simulink model "RC_model_iden"  (R2023b)
settings: Solver=ode1  StartTime=0.0  StopTime=0.848  FixedStep=0.001  RelTol=1e-3  EnableMultiTasking=on
values from neighbouring files (symbols this model uses):
  a = 0.3    [RC_cal_demo.m]    (also in RC_cal_demo_01.m = 1.19001595204e-05; RC_cal_dongtai.m = 4.75514899903e-06; RC_iden_demo.m = V(1); RC_iden_demo01.m = V(1))
  a1 = 189.2    [RC_cal_demo.m]    (also in RC_cal_demo_01.m = 216.986140272; RC_iden_demo.m = V(2); RC_iden_demo01.m = V(2); RC_iden_dongtai.m = 0)
  a2 = 709.081    [RC_cal_demo.m]    (also in RC_cal_demo_01.m = 51.9969921477; RC_iden_demo.m = V(3); RC_iden_demo01.m = V(3); RC_iden_dongtai.m = 0)
  a3 = 0    [RC_cal_demo.m]    (also in RC_cal_demo_01.m = -4.85038740997; RC_cal_dongtai.m = -4.66745370581; RC_iden_demo.m = V(4); RC_iden_demo01.m = V(4))
  b = 0    [RC_cal_demo.m]    (also in RC_cal_demo_01.m = -4.99998404294; RC_cal_dongtai.m = -5.74572134537; RC_iden_Optimization_fmincon_11canshu.m = []; RC_iden_Optimization_fmincon_dongtai.m = [])
  c1 = 11    [RC_cal_demo.m]    (also in RC_cal_demo_01.m = 3.69821992975; RC_iden_demo.m = V(6); RC_iden_demo01.m = V(6); RC_iden_dongtai.m = 0)
  c2 = 22.7    [RC_cal_demo.m]    (also in RC_cal_demo_01.m = 8.28628350298; RC_iden_demo.m = V(7); RC_iden_demo01.m = V(7); RC_iden_dongtai.m = 0)
  c3 = 0    [RC_cal_demo.m]    (also in RC_cal_demo_01.m = 0.0112779556916; RC_iden_demo.m = V(8); RC_iden_demo01.m = V(8); RC_iden_dongtai.m = V(4))
  f0 = -2.1    [RC_cal_demo.m]    (also in RC_cal_demo_01.m = 4.66079282314; RC_cal_dongtai.m = 4.52749017489; RC_iden_demo.m = V(9); RC_iden_demo01.m = V(9))
  k = 0.3    [RC_cal_demo.m]    (also in RC_cal_demo_01.m = -0.0271829954254; RC_cal_dongtai.m = -0.017999550541; RC_iden_demo.m = V(10); RC_iden_demo01.m = V(10))
  m = 0.0141707256428496    (= 0.0141707256428)    [RC_cal_demo_01.m]    (also in RC_cal_dongtai.m = 0.0195846403036; RC_iden_demo01.m = V(11); RC_iden_dongtai.m = V(7))
settings Model: Creator=lenovo  LastModifiedBy=Lenovo
settings SolverCC: AlgebraicLoopSolver=TrustRegion
settings DataIOCC: ReturnWorkspaceOutputs=off
settings OptimizationCC: LifeSpan=inf
settings DebuggingCC: UnconnectedInputMsg=warning  UnconnectedOutputMsg=warning  UnconnectedLineMsg=warning  SFUnexpectedBacktrackingDiag=warning  SFNoUnconditionalDefaultTransitionDiag=warning  SFExecutionAtInitializationDiag=none  ArithmeticOperatorsInVariantConditions=warning
settings ModelReferenceCC: EnableRefExpFcnMdlSchedulingChecks=on
settings SFSimCC: SimUseLocalCustomCode=off  CustomCodeUndefinedFunction=UseInterfaceOnly
settings RTWCC: RTWUseLocalCustomCode=off
settings CodeAppCC: StateflowObjectComments=on
settings GRTTargetCC: TargetLangStandard=C89/C90 (ANSI)
settings ConfigComp: CovMetricSettings=dw  CovSaveCumulativeToWorkspaceVar=on  CovSaveSingleToWorkspaceVar=on  CovExternalEMLEnable=off

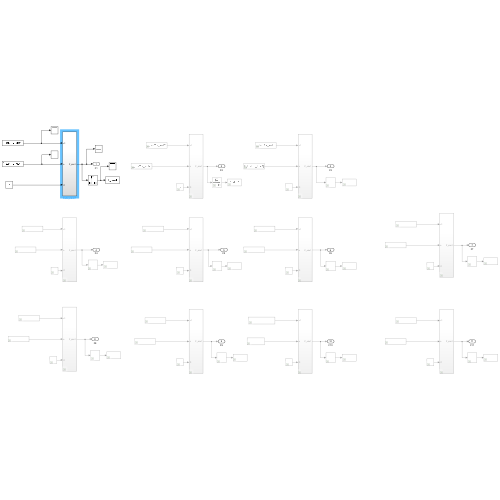
[thumbnail: Simulink's stored preview of the top-level diagram]
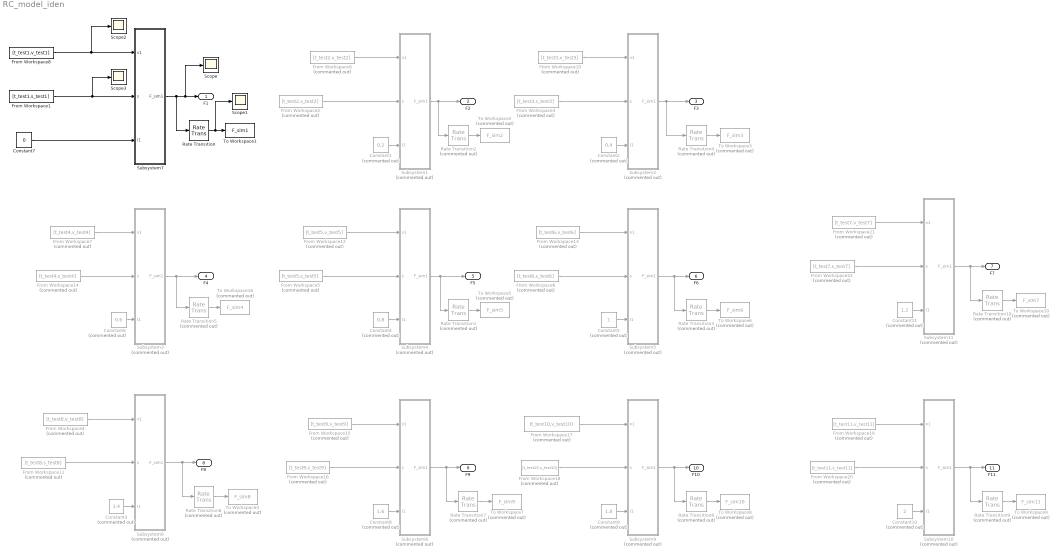
== system RC_model_iden ==
  Constant1 : Constant  Commented=on  Value=0.2
  Constant10 : Constant  Commented=on  Value=2
  Constant11 : Constant  Commented=on  Value=1.2
  Constant2 : Constant  Commented=on  Value=0.4
  Constant3 : Constant  Commented=on  Value=1.4
  Constant4 : Constant  Commented=on  Value=0.8
  Constant5 : Constant  Commented=on
  Constant6 : Constant  Commented=on  Value=0.6
  Constant7 : Constant  Value=0
  Constant8 : Constant  Commented=on  Value=1.6
  Constant9 : Constant  Commented=on  Value=1.8
  From Workspace1 : FromWorkspace  VariableName=[t_test1,s_test1]
  From Workspace10 : FromWorkspace  Commented=on  VariableName=[t_test3,v_test3]
  From Workspace11 : FromWorkspace  Commented=on  VariableName=[t_test8,s_test8]
  From Workspace12 : FromWorkspace  Commented=on  VariableName=[t_test5,v_test5]
  From Workspace13 : FromWorkspace  Commented=on  VariableName=[t_test6,v_test6]
  From Workspace14 : FromWorkspace  Commented=on  VariableName=[t_test4,s_test4]
  From Workspace15 : FromWorkspace  Commented=on  VariableName=[t_test9,v_test9]
  From Workspace16 : FromWorkspace  Commented=on  VariableName=[t_test9,s_test9]
  From Workspace17 : FromWorkspace  Commented=on  VariableName=[t_test10,v_test10]
  From Workspace18 : FromWorkspace  Commented=on  VariableName=[t_test10,s_test10]
  From Workspace19 : FromWorkspace  Commented=on  VariableName=[t_test11,v_test11]
  From Workspace2 : FromWorkspace  Commented=on  VariableName=[t_test2,s_test2]
  From Workspace20 : FromWorkspace  Commented=on  VariableName=[t_test11,s_test11]
  From Workspace21 : FromWorkspace  Commented=on  VariableName=[t_test7,v_test7]
  From Workspace22 : FromWorkspace  Commented=on  VariableName=[t_test7,s_test7]
  From Workspace3 : FromWorkspace  Commented=on  VariableName=[t_test3,s_test3]
  From Workspace4 : FromWorkspace  Commented=on  VariableName=[t_test8,v_test8]
  From Workspace5 : FromWorkspace  Commented=on  VariableName=[t_test5,s_test5]
  From Workspace6 : FromWorkspace  Commented=on  VariableName=[t_test6,s_test6]
  From Workspace7 : FromWorkspace  Commented=on  VariableName=[t_test4,v_test4]
  From Workspace8 : FromWorkspace  VariableName=[t_test1,v_test1]
  From Workspace9 : FromWorkspace  Commented=on  VariableName=[t_test2,v_test2]
  Rate Transition : RateTransition  OutPortSampleTime=0.001
  Rate Transition{1..10} (10 alike) : RateTransition  Commented=on  OutPortSampleTime=0.001
  Scope{,1..3} (4 alike) : Scope
  Subsystem1 : Subsystem  Commented=on
  Subsystem10 : Subsystem  Commented=on
  Subsystem11 : Subsystem  Commented=on
  Subsystem2 : Subsystem  Commented=on
  Subsystem3 : Subsystem  Commented=on
  Subsystem4 : Subsystem  Commented=on
  Subsystem5 : Subsystem  Commented=on
  Subsystem6 : Subsystem  Commented=on
  Subsystem7 : Subsystem
  Subsystem8 : Subsystem  Commented=on
  Subsystem9 : Subsystem  Commented=on
  To Workspace1 : ToWorkspace  VariableName=F_sim1  SampleTime=-1
  To Workspace10 : ToWorkspace  Commented=on  VariableName=F_sim7  SampleTime=-1
  To Workspace16 : ToWorkspace  Commented=on  VariableName=F_sim4  SampleTime=-1
  To Workspace2 : ToWorkspace  Commented=on  VariableName=F_sim2  SampleTime=-1
  To Workspace3 : ToWorkspace  Commented=on  VariableName=F_sim3  SampleTime=-1
  To Workspace4 : ToWorkspace  Commented=on  VariableName=F_sim8  SampleTime=-1
  To Workspace5 : ToWorkspace  Commented=on  VariableName=F_sim5  SampleTime=-1
  To Workspace6 : ToWorkspace  Commented=on  VariableName=F_sim6  SampleTime=-1
  To Workspace7 : ToWorkspace  Commented=on  VariableName=F_sim9  SampleTime=-1
  To Workspace8 : ToWorkspace  Commented=on  VariableName=F_sim10  SampleTime=-1
  To Workspace9 : ToWorkspace  Commented=on  VariableName=F_sim11  SampleTime=-1
  F1 : Outport  VectorParamsAs1DForOutWhenUnconnected=off
  F2 : Outport  Port=2  VectorParamsAs1DForOutWhenUnconnected=off
  F3 : Outport  Port=3  VectorParamsAs1DForOutWhenUnconnected=off
  F4 : Outport  Port=4  VectorParamsAs1DForOutWhenUnconnected=off
  F5 : Outport  Port=5  VectorParamsAs1DForOutWhenUnconnected=off
  F6 : Outport  Port=6  VectorParamsAs1DForOutWhenUnconnected=off
  F7 : Outport  Port=7  VectorParamsAs1DForOutWhenUnconnected=off
  F8 : Outport  Port=8  VectorParamsAs1DForOutWhenUnconnected=off
  F9 : Outport  Port=9  VectorParamsAs1DForOutWhenUnconnected=off
  F10 : Outport  Port=10  VectorParamsAs1DForOutWhenUnconnected=off
  F11 : Outport  Port=11  VectorParamsAs1DForOutWhenUnconnected=off
  wires:
  From Workspace9/1 -> Subsystem1/1(v1)
  Subsystem1/1(F_sim1) -> F2/1, Rate Transition2/1
  From Workspace2/1 -> Subsystem1/2(s)
  Constant1/1 -> Subsystem1/3(I1)
  From Workspace10/1 -> Subsystem2/1(v1)
  Subsystem2/1(F_sim1) -> Rate Transition4/1, F3/1
  From Workspace3/1 -> Subsystem2/2(s)
  Constant2/1 -> Subsystem2/3(I1)
  From Workspace12/1 -> Subsystem4/1(v1)
  Subsystem4/1(F_sim1) -> F5/1, Rate Transition1/1
  From Workspace5/1 -> Subsystem4/2(s)
  Constant4/1 -> Subsystem4/3(I1)
  From Workspace13/1 -> Subsystem5/1(v1)
  Subsystem5/1(F_sim1) -> Rate Transition3/1, F6/1
  From Workspace6/1 -> Subsystem5/2(s)
  Constant5/1 -> Subsystem5/3(I1)
  From Workspace8/1 -> Scope2/1, Subsystem7/1(v1)
  Subsystem7/1(F_sim1) -> Rate Transition/1, Scope/1, F1/1
  From Workspace1/1 -> Scope3/1, Subsystem7/2(s)
  Constant7/1 -> Subsystem7/3(I1)
  Rate Transition/1 -> To Workspace1/1, Scope1/1
  Rate Transition1/1 -> To Workspace5/1
  Rate Transition2/1 -> To Workspace2/1
  Rate Transition3/1 -> To Workspace6/1
  Rate Transition4/1 -> To Workspace3/1
  Rate Transition5/1 -> To Workspace16/1
  Constant6/1 -> Subsystem3/3(I1)
  From Workspace14/1 -> Subsystem3/2(s)
  Subsystem3/1(F_sim1) -> F4/1, Rate Transition5/1
  From Workspace7/1 -> Subsystem3/1(v1)
  Rate Transition6/1 -> To Workspace4/1
  From Workspace11/1 -> Subsystem6/2(s)
  Constant3/1 -> Subsystem6/3(I1)
  From Workspace4/1 -> Subsystem6/1(v1)
  Subsystem6/1(F_sim1) -> Rate Transition6/1, F8/1
  Rate Transition7/1 -> To Workspace7/1
  From Workspace16/1 -> Subsystem8/2(s)
  Constant8/1 -> Subsystem8/3(I1)
  From Workspace15/1 -> Subsystem8/1(v1)
  Subsystem8/1(F_sim1) -> Rate Transition7/1, F9/1
  Rate Transition8/1 -> To Workspace8/1
  From Workspace18/1 -> Subsystem9/2(s)
  Constant9/1 -> Subsystem9/3(I1)
  From Workspace17/1 -> Subsystem9/1(v1)
  Subsystem9/1(F_sim1) -> Rate Transition8/1, F10/1
  Rate Transition9/1 -> To Workspace9/1
  From Workspace20/1 -> Subsystem10/2(s)
  Constant10/1 -> Subsystem10/3(I1)
  From Workspace19/1 -> Subsystem10/1(v1)
  Subsystem10/1(F_sim1) -> Rate Transition9/1, F11/1
  Rate Transition10/1 -> To Workspace10/1
  From Workspace22/1 -> Subsystem11/2(s)
  Constant11/1 -> Subsystem11/3(I1)
  From Workspace21/1 -> Subsystem11/1(v1)
  Subsystem11/1(F_sim1) -> Rate Transition10/1, F7/1

== system RC_model_iden/Subsystem1 ==
  v1 : Inport
  s : Inport  Port=2
  I1 : Inport  Port=3
  Ftra : Subsystem
  Subsystem : Subsystem
  F_sim1 : Outport  VectorParamsAs1DForOutWhenUnconnected=off
  wires:
  s/1 -> Ftra/2(x1), Subsystem/1(x1)
  v1/1 -> Ftra/3(x2)
  I1/1 -> Ftra/1(I)
  Subsystem/1(z) -> Ftra/4(z)
  Ftra/1(Ftra) -> F_sim1/1

== system RC_model_iden/Subsystem10 ==
  v1 : Inport
  s : Inport  Port=2
  I1 : Inport  Port=3
  Ftra : Subsystem
  Subsystem : Subsystem
  F_sim1 : Outport  VectorParamsAs1DForOutWhenUnconnected=off
  wires:
  s/1 -> Ftra/2(x1), Subsystem/1(x1)
  v1/1 -> Ftra/3(x2)
  I1/1 -> Ftra/1(I)
  Subsystem/1(z) -> Ftra/4(z)
  Ftra/1(Ftra) -> F_sim1/1

== system RC_model_iden/Subsystem11 ==
  v1 : Inport
  s : Inport  Port=2
  I1 : Inport  Port=3
  Ftra : Subsystem
  Subsystem : Subsystem
  F_sim1 : Outport  VectorParamsAs1DForOutWhenUnconnected=off
  wires:
  s/1 -> Ftra/2(x1), Subsystem/1(x1)
  v1/1 -> Ftra/3(x2)
  I1/1 -> Ftra/1(I)
  Subsystem/1(z) -> Ftra/4(z)
  Ftra/1(Ftra) -> F_sim1/1

== system RC_model_iden/Subsystem2 ==
  v1 : Inport
  s : Inport  Port=2
  I1 : Inport  Port=3
  Ftra : Subsystem
  Subsystem : Subsystem
  F_sim1 : Outport  VectorParamsAs1DForOutWhenUnconnected=off
  wires:
  s/1 -> Ftra/2(x1), Subsystem/1(x1)
  v1/1 -> Ftra/3(x2)
  I1/1 -> Ftra/1(I)
  Subsystem/1(z) -> Ftra/4(z)
  Ftra/1(Ftra) -> F_sim1/1

== system RC_model_iden/Subsystem3 ==
  v1 : Inport
  s : Inport  Port=2
  I1 : Inport  Port=3
  Ftra : Subsystem
  Subsystem : Subsystem
  F_sim1 : Outport  VectorParamsAs1DForOutWhenUnconnected=off
  wires:
  s/1 -> Ftra/2(x1), Subsystem/1(x1)
  v1/1 -> Ftra/3(x2)
  I1/1 -> Ftra/1(I)
  Subsystem/1(z) -> Ftra/4(z)
  Ftra/1(Ftra) -> F_sim1/1

== system RC_model_iden/Subsystem4 ==
  v1 : Inport
  s : Inport  Port=2
  I1 : Inport  Port=3
  Ftra : Subsystem
  Subsystem : Subsystem
  F_sim1 : Outport  VectorParamsAs1DForOutWhenUnconnected=off
  wires:
  s/1 -> Ftra/2(x1), Subsystem/1(x1)
  v1/1 -> Ftra/3(x2)
  I1/1 -> Ftra/1(I)
  Subsystem/1(z) -> Ftra/4(z)
  Ftra/1(Ftra) -> F_sim1/1

== system RC_model_iden/Subsystem5 ==
  v1 : Inport
  s : Inport  Port=2
  I1 : Inport  Port=3
  Ftra : Subsystem
  Subsystem : Subsystem
  F_sim1 : Outport  VectorParamsAs1DForOutWhenUnconnected=off
  wires:
  s/1 -> Ftra/2(x1), Subsystem/1(x1)
  v1/1 -> Ftra/3(x2)
  I1/1 -> Ftra/1(I)
  Subsystem/1(z) -> Ftra/4(z)
  Ftra/1(Ftra) -> F_sim1/1

== system RC_model_iden/Subsystem6 ==
  v1 : Inport
  s : Inport  Port=2
  I1 : Inport  Port=3
  Ftra : Subsystem
  Subsystem : Subsystem
  F_sim1 : Outport  VectorParamsAs1DForOutWhenUnconnected=off
  wires:
  s/1 -> Ftra/2(x1), Subsystem/1(x1)
  v1/1 -> Ftra/3(x2)
  I1/1 -> Ftra/1(I)
  Subsystem/1(z) -> Ftra/4(z)
  Ftra/1(Ftra) -> F_sim1/1

== system RC_model_iden/Subsystem7 ==
  v1 : Inport
  s : Inport  Port=2
  I1 : Inport  Port=3
  Ftra : Subsystem
  Subsystem : Subsystem
  F_sim1 : Outport  VectorParamsAs1DForOutWhenUnconnected=off
  wires:
  s/1 -> Ftra/2(x1), Subsystem/1(x1)
  v1/1 -> Subsystem/2(v1), Ftra/3(x2)
  I1/1 -> Ftra/1(I)
  Subsystem/1(z) -> Ftra/4(z)
  Ftra/1(Ftra) -> F_sim1/1

== system RC_model_iden/Subsystem8 ==
  v1 : Inport
  s : Inport  Port=2
  I1 : Inport  Port=3
  Ftra : Subsystem
  Subsystem : Subsystem
  F_sim1 : Outport  VectorParamsAs1DForOutWhenUnconnected=off
  wires:
  s/1 -> Ftra/2(x1), Subsystem/1(x1)
  v1/1 -> Ftra/3(x2)
  I1/1 -> Ftra/1(I)
  Subsystem/1(z) -> Ftra/4(z)
  Ftra/1(Ftra) -> F_sim1/1

== system RC_model_iden/Subsystem9 ==
  v1 : Inport
  s : Inport  Port=2
  I1 : Inport  Port=3
  Ftra : Subsystem
  Subsystem : Subsystem
  F_sim1 : Outport  VectorParamsAs1DForOutWhenUnconnected=off
  wires:
  s/1 -> Ftra/2(x1), Subsystem/1(x1)
  v1/1 -> Ftra/3(x2)
  I1/1 -> Ftra/1(I)
  Subsystem/1(z) -> Ftra/4(z)
  Ftra/1(Ftra) -> F_sim1/1

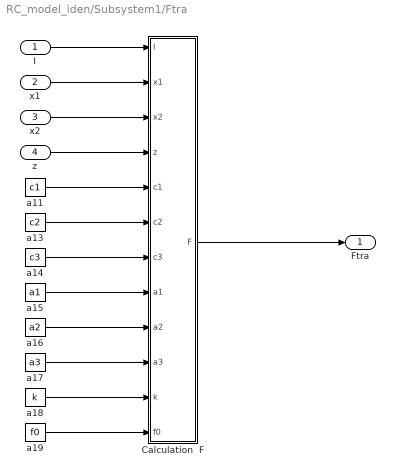
== system RC_model_iden/Subsystem1/Ftra ==
  I : Inport
  x1 : Inport  Port=2
  x2 : Inport  Port=3
  z : Inport  Port=4
  Calculation  F : MATLAB Function  TreatAsAtomicUnit=on
  a11 : Constant  Value=c1  SampleTime=-1
  a13 : Constant  Value=c2  SampleTime=-1
  a14 : Constant  Value=c3  SampleTime=-1
  a15 : Constant  Value=a1  SampleTime=-1
  a16 : Constant  Value=a2  SampleTime=-1
  a17 : Constant  Value=a3  SampleTime=-1
  a18 : Constant  Value=k  SampleTime=-1
  a19 : Constant  Value=f0  SampleTime=-1
  Ftra : Outport  VectorParamsAs1DForOutWhenUnconnected=off
  wires:
  x2/1 -> Calculation  F/3(x2)
  a14/1 -> Calculation  F/7(c3)
  a15/1 -> Calculation  F/8(a1)
  a16/1 -> Calculation  F/9(a2)
  a17/1 -> Calculation  F/10(a3)
  a19/1 -> Calculation  F/12(f0)
  a18/1 -> Calculation  F/11(k)
  a13/1 -> Calculation  F/6(c2)
  a11/1 -> Calculation  F/5(c1)
  Calculation  F/1(F) -> Ftra/1
  z/1 -> Calculation  F/4(z)
  x1/1 -> Calculation  F/2(x1)
  I/1 -> Calculation  F/1(I)

== system RC_model_iden/Subsystem1/Subsystem ==
  x1 : Inport
  Constant : Constant  Value=a
  Constant1 : Constant  Value=b
  Delay : Delay  DelayLength=1  InitialCondition=0
  Delay1 : Delay  DelayLength=1  InitialCondition=0
  Delay2 : Delay  DelayLength=1  InitialCondition=0.17
  Delay3 : Delay  DelayLength=1  InitialCondition=0
  MATLAB Function : MATLAB Function  TreatAsAtomicUnit=on
  z : Outport  VectorParamsAs1DForOutWhenUnconnected=off
  wires:
  Delay3/1 -> MATLAB Function/6(x0)
  MATLAB Function/3(x01) -> Delay3/1
  Delay2/1 -> MATLAB Function/7(S0)
  MATLAB Function/4(S01) -> Delay2/1
  Delay1/1 -> MATLAB Function/5(x1k1)
  MATLAB Function/2(x1k2) -> Delay1/1
  Delay/1 -> MATLAB Function/4(zk1)
  MATLAB Function/1(zk) -> z/1, Delay/1
  Constant1/1 -> MATLAB Function/2(b)
  Constant/1 -> MATLAB Function/1(a)
  x1/1 -> MATLAB Function/3(x1k)

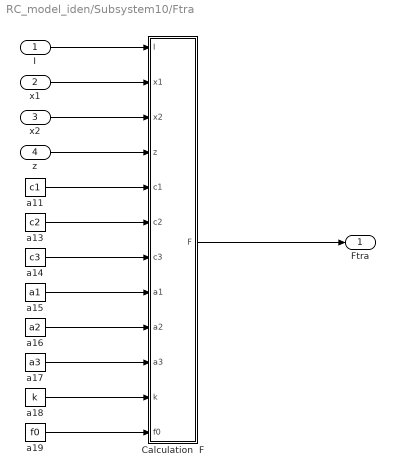
== system RC_model_iden/Subsystem10/Ftra ==
  I : Inport
  x1 : Inport  Port=2
  x2 : Inport  Port=3
  z : Inport  Port=4
  Calculation  F : MATLAB Function  TreatAsAtomicUnit=on
  a11 : Constant  Value=c1  SampleTime=-1
  a13 : Constant  Value=c2  SampleTime=-1
  a14 : Constant  Value=c3  SampleTime=-1
  a15 : Constant  Value=a1  SampleTime=-1
  a16 : Constant  Value=a2  SampleTime=-1
  a17 : Constant  Value=a3  SampleTime=-1
  a18 : Constant  Value=k  SampleTime=-1
  a19 : Constant  Value=f0  SampleTime=-1
  Ftra : Outport  VectorParamsAs1DForOutWhenUnconnected=off
  wires:
  x2/1 -> Calculation  F/3(x2)
  a14/1 -> Calculation  F/7(c3)
  a15/1 -> Calculation  F/8(a1)
  a16/1 -> Calculation  F/9(a2)
  a17/1 -> Calculation  F/10(a3)
  a19/1 -> Calculation  F/12(f0)
  a18/1 -> Calculation  F/11(k)
  a13/1 -> Calculation  F/6(c2)
  a11/1 -> Calculation  F/5(c1)
  Calculation  F/1(F) -> Ftra/1
  z/1 -> Calculation  F/4(z)
  x1/1 -> Calculation  F/2(x1)
  I/1 -> Calculation  F/1(I)

== system RC_model_iden/Subsystem10/Subsystem ==
  x1 : Inport
  Constant : Constant  Value=a
  Constant1 : Constant  Value=b
  Delay : Delay  DelayLength=1  InitialCondition=0
  Delay1 : Delay  DelayLength=1  InitialCondition=0
  Delay2 : Delay  DelayLength=1  InitialCondition=0.17
  Delay3 : Delay  DelayLength=1  InitialCondition=0
  MATLAB Function : MATLAB Function  TreatAsAtomicUnit=on
  z : Outport  VectorParamsAs1DForOutWhenUnconnected=off
  wires:
  Delay3/1 -> MATLAB Function/6(x0)
  MATLAB Function/3(x01) -> Delay3/1
  Delay2/1 -> MATLAB Function/7(S0)
  MATLAB Function/4(S01) -> Delay2/1
  Delay1/1 -> MATLAB Function/5(x1k1)
  MATLAB Function/2(x1k2) -> Delay1/1
  Delay/1 -> MATLAB Function/4(zk1)
  MATLAB Function/1(zk) -> z/1, Delay/1
  Constant1/1 -> MATLAB Function/2(b)
  Constant/1 -> MATLAB Function/1(a)
  x1/1 -> MATLAB Function/3(x1k)

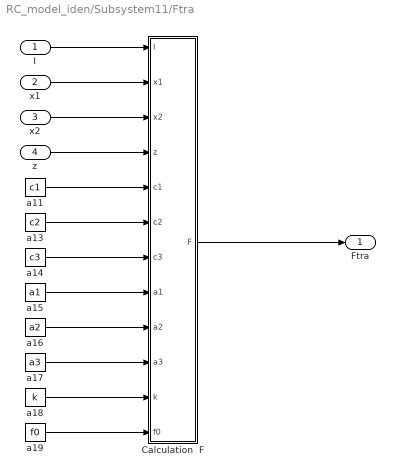
== system RC_model_iden/Subsystem11/Ftra ==
  I : Inport
  x1 : Inport  Port=2
  x2 : Inport  Port=3
  z : Inport  Port=4
  Calculation  F : MATLAB Function  TreatAsAtomicUnit=on
  a11 : Constant  Value=c1  SampleTime=-1
  a13 : Constant  Value=c2  SampleTime=-1
  a14 : Constant  Value=c3  SampleTime=-1
  a15 : Constant  Value=a1  SampleTime=-1
  a16 : Constant  Value=a2  SampleTime=-1
  a17 : Constant  Value=a3  SampleTime=-1
  a18 : Constant  Value=k  SampleTime=-1
  a19 : Constant  Value=f0  SampleTime=-1
  Ftra : Outport  VectorParamsAs1DForOutWhenUnconnected=off
  wires:
  x2/1 -> Calculation  F/3(x2)
  a14/1 -> Calculation  F/7(c3)
  a15/1 -> Calculation  F/8(a1)
  a16/1 -> Calculation  F/9(a2)
  a17/1 -> Calculation  F/10(a3)
  a19/1 -> Calculation  F/12(f0)
  a18/1 -> Calculation  F/11(k)
  a13/1 -> Calculation  F/6(c2)
  a11/1 -> Calculation  F/5(c1)
  Calculation  F/1(F) -> Ftra/1
  z/1 -> Calculation  F/4(z)
  x1/1 -> Calculation  F/2(x1)
  I/1 -> Calculation  F/1(I)

== system RC_model_iden/Subsystem11/Subsystem ==
  x1 : Inport
  Constant : Constant  Value=a
  Constant1 : Constant  Value=b
  Delay : Delay  DelayLength=1  InitialCondition=0
  Delay1 : Delay  DelayLength=1  InitialCondition=0
  Delay2 : Delay  DelayLength=1  InitialCondition=0.17
  Delay3 : Delay  DelayLength=1  InitialCondition=0
  MATLAB Function : MATLAB Function  TreatAsAtomicUnit=on
  z : Outport  VectorParamsAs1DForOutWhenUnconnected=off
  wires:
  Delay3/1 -> MATLAB Function/6(x0)
  MATLAB Function/3(x01) -> Delay3/1
  Delay2/1 -> MATLAB Function/7(S0)
  MATLAB Function/4(S01) -> Delay2/1
  Delay1/1 -> MATLAB Function/5(x1k1)
  MATLAB Function/2(x1k2) -> Delay1/1
  Delay/1 -> MATLAB Function/4(zk1)
  MATLAB Function/1(zk) -> z/1, Delay/1
  Constant1/1 -> MATLAB Function/2(b)
  Constant/1 -> MATLAB Function/1(a)
  x1/1 -> MATLAB Function/3(x1k)

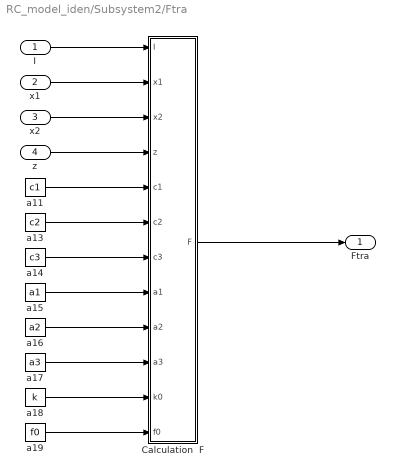
== system RC_model_iden/Subsystem2/Ftra ==
  I : Inport
  x1 : Inport  Port=2
  x2 : Inport  Port=3
  z : Inport  Port=4
  Calculation  F : MATLAB Function  TreatAsAtomicUnit=on
  a11 : Constant  Value=c1  SampleTime=-1
  a13 : Constant  Value=c2  SampleTime=-1
  a14 : Constant  Value=c3  SampleTime=-1
  a15 : Constant  Value=a1  SampleTime=-1
  a16 : Constant  Value=a2  SampleTime=-1
  a17 : Constant  Value=a3  SampleTime=-1
  a18 : Constant  Value=k  SampleTime=-1
  a19 : Constant  Value=f0  SampleTime=-1
  Ftra : Outport  VectorParamsAs1DForOutWhenUnconnected=off
  wires:
  x2/1 -> Calculation  F/3(x2)
  a14/1 -> Calculation  F/7(c3)
  a15/1 -> Calculation  F/8(a1)
  a16/1 -> Calculation  F/9(a2)
  a17/1 -> Calculation  F/10(a3)
  a19/1 -> Calculation  F/12(f0)
  a18/1 -> Calculation  F/11(k0)
  a13/1 -> Calculation  F/6(c2)
  a11/1 -> Calculation  F/5(c1)
  Calculation  F/1(F) -> Ftra/1
  z/1 -> Calculation  F/4(z)
  x1/1 -> Calculation  F/2(x1)
  I/1 -> Calculation  F/1(I)

== system RC_model_iden/Subsystem2/Subsystem ==
  x1 : Inport
  Constant : Constant  Value=a
  Constant1 : Constant  Value=b
  Delay : Delay  DelayLength=1  InitialCondition=0
  Delay1 : Delay  DelayLength=1  InitialCondition=0
  Delay2 : Delay  DelayLength=1  InitialCondition=0.17
  Delay3 : Delay  DelayLength=1  InitialCondition=0
  MATLAB Function : MATLAB Function  TreatAsAtomicUnit=on
  z : Outport  VectorParamsAs1DForOutWhenUnconnected=off
  wires:
  Delay3/1 -> MATLAB Function/6(x0)
  MATLAB Function/3(x01) -> Delay3/1
  Delay2/1 -> MATLAB Function/7(S0)
  MATLAB Function/4(S01) -> Delay2/1
  Delay1/1 -> MATLAB Function/5(x1k1)
  MATLAB Function/2(x1k2) -> Delay1/1
  Delay/1 -> MATLAB Function/4(zk1)
  MATLAB Function/1(zk) -> z/1, Delay/1
  Constant1/1 -> MATLAB Function/2(b)
  Constant/1 -> MATLAB Function/1(a)
  x1/1 -> MATLAB Function/3(x1k)

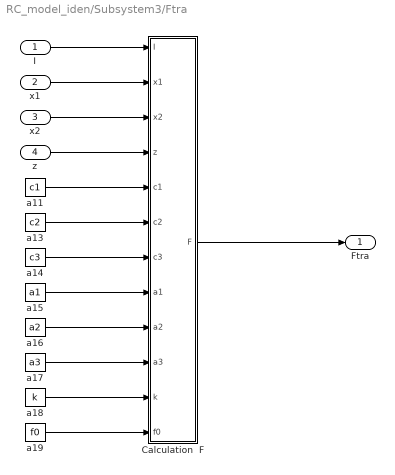
== system RC_model_iden/Subsystem3/Ftra ==
  I : Inport
  x1 : Inport  Port=2
  x2 : Inport  Port=3
  z : Inport  Port=4
  Calculation  F : MATLAB Function  TreatAsAtomicUnit=on
  a11 : Constant  Value=c1  SampleTime=-1
  a13 : Constant  Value=c2  SampleTime=-1
  a14 : Constant  Value=c3  SampleTime=-1
  a15 : Constant  Value=a1  SampleTime=-1
  a16 : Constant  Value=a2  SampleTime=-1
  a17 : Constant  Value=a3  SampleTime=-1
  a18 : Constant  Value=k  SampleTime=-1
  a19 : Constant  Value=f0  SampleTime=-1
  Ftra : Outport  VectorParamsAs1DForOutWhenUnconnected=off
  wires:
  x2/1 -> Calculation  F/3(x2)
  a14/1 -> Calculation  F/7(c3)
  a15/1 -> Calculation  F/8(a1)
  a16/1 -> Calculation  F/9(a2)
  a17/1 -> Calculation  F/10(a3)
  a19/1 -> Calculation  F/12(f0)
  a18/1 -> Calculation  F/11(k)
  a13/1 -> Calculation  F/6(c2)
  a11/1 -> Calculation  F/5(c1)
  Calculation  F/1(F) -> Ftra/1
  z/1 -> Calculation  F/4(z)
  x1/1 -> Calculation  F/2(x1)
  I/1 -> Calculation  F/1(I)

== system RC_model_iden/Subsystem3/Subsystem ==
  x1 : Inport
  Constant : Constant  Value=a
  Constant1 : Constant  Value=b
  Delay : Delay  DelayLength=1  InitialCondition=0
  Delay1 : Delay  DelayLength=1  InitialCondition=0
  Delay2 : Delay  DelayLength=1  InitialCondition=0.17
  Delay3 : Delay  DelayLength=1  InitialCondition=0
  MATLAB Function : MATLAB Function  TreatAsAtomicUnit=on
  z : Outport  VectorParamsAs1DForOutWhenUnconnected=off
  wires:
  Delay3/1 -> MATLAB Function/6(x0)
  MATLAB Function/3(x01) -> Delay3/1
  Delay2/1 -> MATLAB Function/7(S0)
  MATLAB Function/4(S01) -> Delay2/1
  Delay1/1 -> MATLAB Function/5(x1k1)
  MATLAB Function/2(x1k2) -> Delay1/1
  Delay/1 -> MATLAB Function/4(zk1)
  MATLAB Function/1(zk) -> z/1, Delay/1
  Constant1/1 -> MATLAB Function/2(b)
  Constant/1 -> MATLAB Function/1(a)
  x1/1 -> MATLAB Function/3(x1k)

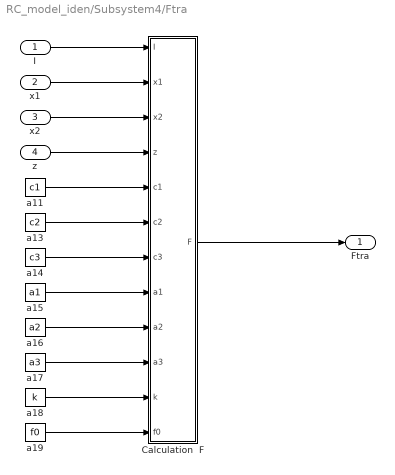
== system RC_model_iden/Subsystem4/Ftra ==
  I : Inport
  x1 : Inport  Port=2
  x2 : Inport  Port=3
  z : Inport  Port=4
  Calculation  F : MATLAB Function  TreatAsAtomicUnit=on
  a11 : Constant  Value=c1  SampleTime=-1
  a13 : Constant  Value=c2  SampleTime=-1
  a14 : Constant  Value=c3  SampleTime=-1
  a15 : Constant  Value=a1  SampleTime=-1
  a16 : Constant  Value=a2  SampleTime=-1
  a17 : Constant  Value=a3  SampleTime=-1
  a18 : Constant  Value=k  SampleTime=-1
  a19 : Constant  Value=f0  SampleTime=-1
  Ftra : Outport  VectorParamsAs1DForOutWhenUnconnected=off
  wires:
  x2/1 -> Calculation  F/3(x2)
  a14/1 -> Calculation  F/7(c3)
  a15/1 -> Calculation  F/8(a1)
  a16/1 -> Calculation  F/9(a2)
  a17/1 -> Calculation  F/10(a3)
  a19/1 -> Calculation  F/12(f0)
  a18/1 -> Calculation  F/11(k)
  a13/1 -> Calculation  F/6(c2)
  a11/1 -> Calculation  F/5(c1)
  Calculation  F/1(F) -> Ftra/1
  z/1 -> Calculation  F/4(z)
  x1/1 -> Calculation  F/2(x1)
  I/1 -> Calculation  F/1(I)

== system RC_model_iden/Subsystem4/Subsystem ==
  x1 : Inport
  Constant : Constant  Value=a
  Constant1 : Constant  Value=b
  Delay : Delay  DelayLength=1  InitialCondition=0
  Delay1 : Delay  DelayLength=1  InitialCondition=0
  Delay2 : Delay  DelayLength=1  InitialCondition=0.17
  Delay3 : Delay  DelayLength=1  InitialCondition=0
  MATLAB Function : MATLAB Function  TreatAsAtomicUnit=on
  z : Outport  VectorParamsAs1DForOutWhenUnconnected=off
  wires:
  Delay3/1 -> MATLAB Function/6(x0)
  MATLAB Function/3(x01) -> Delay3/1
  Delay2/1 -> MATLAB Function/7(S0)
  MATLAB Function/4(S01) -> Delay2/1
  Delay1/1 -> MATLAB Function/5(x1k1)
  MATLAB Function/2(x1k2) -> Delay1/1
  Delay/1 -> MATLAB Function/4(zk1)
  MATLAB Function/1(zk) -> z/1, Delay/1
  Constant1/1 -> MATLAB Function/2(b)
  Constant/1 -> MATLAB Function/1(a)
  x1/1 -> MATLAB Function/3(x1k)

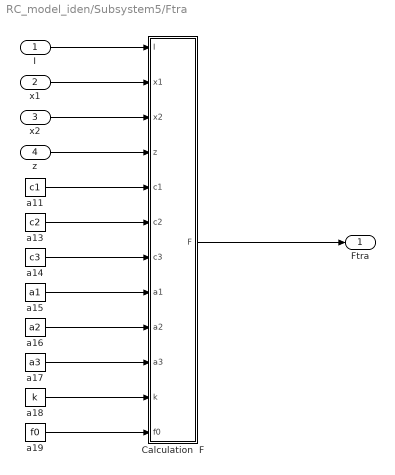
== system RC_model_iden/Subsystem5/Ftra ==
  I : Inport
  x1 : Inport  Port=2
  x2 : Inport  Port=3
  z : Inport  Port=4
  Calculation  F : MATLAB Function  TreatAsAtomicUnit=on
  a11 : Constant  Value=c1  SampleTime=-1
  a13 : Constant  Value=c2  SampleTime=-1
  a14 : Constant  Value=c3  SampleTime=-1
  a15 : Constant  Value=a1  SampleTime=-1
  a16 : Constant  Value=a2  SampleTime=-1
  a17 : Constant  Value=a3  SampleTime=-1
  a18 : Constant  Value=k  SampleTime=-1
  a19 : Constant  Value=f0  SampleTime=-1
  Ftra : Outport  VectorParamsAs1DForOutWhenUnconnected=off
  wires:
  x2/1 -> Calculation  F/3(x2)
  a14/1 -> Calculation  F/7(c3)
  a15/1 -> Calculation  F/8(a1)
  a16/1 -> Calculation  F/9(a2)
  a17/1 -> Calculation  F/10(a3)
  a19/1 -> Calculation  F/12(f0)
  a18/1 -> Calculation  F/11(k)
  a13/1 -> Calculation  F/6(c2)
  a11/1 -> Calculation  F/5(c1)
  Calculation  F/1(F) -> Ftra/1
  z/1 -> Calculation  F/4(z)
  x1/1 -> Calculation  F/2(x1)
  I/1 -> Calculation  F/1(I)

== system RC_model_iden/Subsystem5/Subsystem ==
  x1 : Inport
  Constant : Constant  Value=a
  Constant1 : Constant  Value=b
  Delay : Delay  DelayLength=1  InitialCondition=0
  Delay1 : Delay  DelayLength=1  InitialCondition=0
  Delay2 : Delay  DelayLength=1  InitialCondition=0.17
  Delay3 : Delay  DelayLength=1  InitialCondition=0
  MATLAB Function : MATLAB Function  TreatAsAtomicUnit=on
  z : Outport  VectorParamsAs1DForOutWhenUnconnected=off
  wires:
  Delay3/1 -> MATLAB Function/6(x0)
  MATLAB Function/3(x01) -> Delay3/1
  Delay2/1 -> MATLAB Function/7(S0)
  MATLAB Function/4(S01) -> Delay2/1
  Delay1/1 -> MATLAB Function/5(x1k1)
  MATLAB Function/2(x1k2) -> Delay1/1
  Delay/1 -> MATLAB Function/4(zk1)
  MATLAB Function/1(zk) -> z/1, Delay/1
  Constant1/1 -> MATLAB Function/2(b)
  Constant/1 -> MATLAB Function/1(a)
  x1/1 -> MATLAB Function/3(x1k)

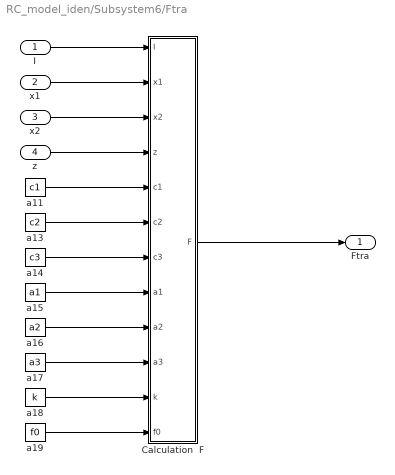
== system RC_model_iden/Subsystem6/Ftra ==
  I : Inport
  x1 : Inport  Port=2
  x2 : Inport  Port=3
  z : Inport  Port=4
  Calculation  F : MATLAB Function  TreatAsAtomicUnit=on
  a11 : Constant  Value=c1  SampleTime=-1
  a13 : Constant  Value=c2  SampleTime=-1
  a14 : Constant  Value=c3  SampleTime=-1
  a15 : Constant  Value=a1  SampleTime=-1
  a16 : Constant  Value=a2  SampleTime=-1
  a17 : Constant  Value=a3  SampleTime=-1
  a18 : Constant  Value=k  SampleTime=-1
  a19 : Constant  Value=f0  SampleTime=-1
  Ftra : Outport  VectorParamsAs1DForOutWhenUnconnected=off
  wires:
  x2/1 -> Calculation  F/3(x2)
  a14/1 -> Calculation  F/7(c3)
  a15/1 -> Calculation  F/8(a1)
  a16/1 -> Calculation  F/9(a2)
  a17/1 -> Calculation  F/10(a3)
  a19/1 -> Calculation  F/12(f0)
  a18/1 -> Calculation  F/11(k)
  a13/1 -> Calculation  F/6(c2)
  a11/1 -> Calculation  F/5(c1)
  Calculation  F/1(F) -> Ftra/1
  z/1 -> Calculation  F/4(z)
  x1/1 -> Calculation  F/2(x1)
  I/1 -> Calculation  F/1(I)

== system RC_model_iden/Subsystem6/Subsystem ==
  x1 : Inport
  Constant : Constant  Value=a
  Constant1 : Constant  Value=b
  Delay : Delay  DelayLength=1  InitialCondition=0
  Delay1 : Delay  DelayLength=1  InitialCondition=0
  Delay2 : Delay  DelayLength=1  InitialCondition=0.17
  Delay3 : Delay  DelayLength=1  InitialCondition=0
  MATLAB Function : MATLAB Function  TreatAsAtomicUnit=on
  z : Outport  VectorParamsAs1DForOutWhenUnconnected=off
  wires:
  Delay3/1 -> MATLAB Function/6(x0)
  MATLAB Function/3(x01) -> Delay3/1
  Delay2/1 -> MATLAB Function/7(S0)
  MATLAB Function/4(S01) -> Delay2/1
  Delay1/1 -> MATLAB Function/5(x1k1)
  MATLAB Function/2(x1k2) -> Delay1/1
  Delay/1 -> MATLAB Function/4(zk1)
  MATLAB Function/1(zk) -> z/1, Delay/1
  Constant1/1 -> MATLAB Function/2(b)
  Constant/1 -> MATLAB Function/1(a)
  x1/1 -> MATLAB Function/3(x1k)

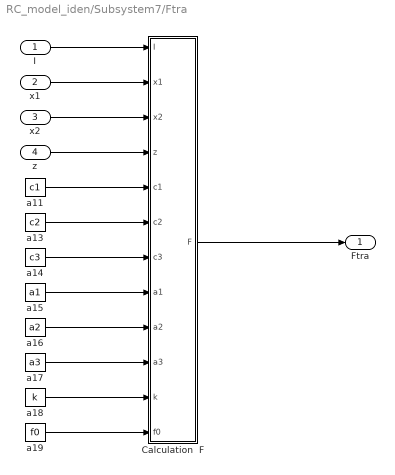
== system RC_model_iden/Subsystem7/Ftra ==
  I : Inport
  x1 : Inport  Port=2
  x2 : Inport  Port=3
  z : Inport  Port=4
  Calculation  F : MATLAB Function  TreatAsAtomicUnit=on
  a11 : Constant  Value=c1  SampleTime=-1
  a13 : Constant  Value=c2  SampleTime=-1
  a14 : Constant  Value=c3  SampleTime=-1
  a15 : Constant  Value=a1  SampleTime=-1
  a16 : Constant  Value=a2  SampleTime=-1
  a17 : Constant  Value=a3  SampleTime=-1
  a18 : Constant  Value=k  SampleTime=-1
  a19 : Constant  Value=f0  SampleTime=-1
  Ftra : Outport  VectorParamsAs1DForOutWhenUnconnected=off
  wires:
  x2/1 -> Calculation  F/3(x2)
  a14/1 -> Calculation  F/7(c3)
  a15/1 -> Calculation  F/8(a1)
  a16/1 -> Calculation  F/9(a2)
  a17/1 -> Calculation  F/10(a3)
  a19/1 -> Calculation  F/12(f0)
  a18/1 -> Calculation  F/11(k)
  a13/1 -> Calculation  F/6(c2)
  a11/1 -> Calculation  F/5(c1)
  Calculation  F/1(F) -> Ftra/1
  z/1 -> Calculation  F/4(z)
  x1/1 -> Calculation  F/2(x1)
  I/1 -> Calculation  F/1(I)

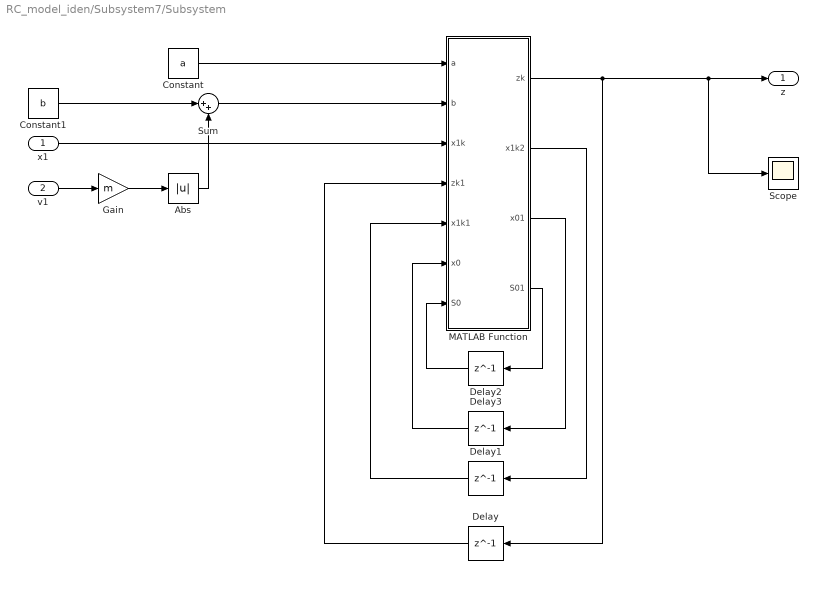
== system RC_model_iden/Subsystem7/Subsystem ==
  x1 : Inport
  v1 : Inport  Port=2
  Abs : Abs  SaturateOnIntegerOverflow=off
  Constant : Constant  Value=a
  Constant1 : Constant  Value=b
  Delay : Delay  DelayLength=1  InitialCondition=0
  Delay1 : Delay  DelayLength=1  InitialCondition=0
  Delay2 : Delay  DelayLength=1  InitialCondition=0.17
  Delay3 : Delay  DelayLength=1  InitialCondition=0
  Gain : Gain  Gain=m
  MATLAB Function : MATLAB Function  TreatAsAtomicUnit=on
  Scope : Scope
  Sum : Sum  Inputs=|++
  z : Outport  VectorParamsAs1DForOutWhenUnconnected=off
  wires:
  Delay3/1 -> MATLAB Function/6(x0)
  MATLAB Function/3(x01) -> Delay3/1
  Delay2/1 -> MATLAB Function/7(S0)
  MATLAB Function/4(S01) -> Delay2/1
  Delay1/1 -> MATLAB Function/5(x1k1)
  MATLAB Function/2(x1k2) -> Delay1/1
  Delay/1 -> MATLAB Function/4(zk1)
  Constant/1 -> MATLAB Function/1(a)
  x1/1 -> MATLAB Function/3(x1k)
  MATLAB Function/1(zk) -> Scope/1, z/1, Delay/1
  Constant1/1 -> Sum/1
  Sum/1 -> MATLAB Function/2(b)
  v1/1 -> Gain/1
  Gain/1 -> Abs/1
  Abs/1 -> Sum/2

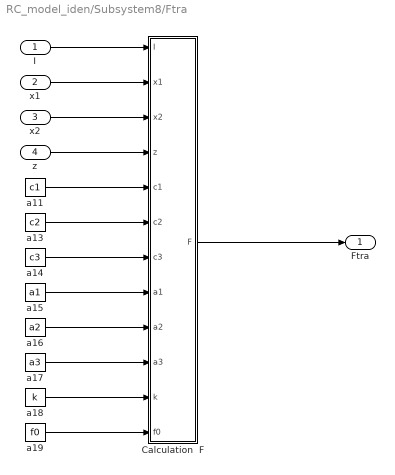
== system RC_model_iden/Subsystem8/Ftra ==
  I : Inport
  x1 : Inport  Port=2
  x2 : Inport  Port=3
  z : Inport  Port=4
  Calculation  F : MATLAB Function  TreatAsAtomicUnit=on
  a11 : Constant  Value=c1  SampleTime=-1
  a13 : Constant  Value=c2  SampleTime=-1
  a14 : Constant  Value=c3  SampleTime=-1
  a15 : Constant  Value=a1  SampleTime=-1
  a16 : Constant  Value=a2  SampleTime=-1
  a17 : Constant  Value=a3  SampleTime=-1
  a18 : Constant  Value=k  SampleTime=-1
  a19 : Constant  Value=f0  SampleTime=-1
  Ftra : Outport  VectorParamsAs1DForOutWhenUnconnected=off
  wires:
  x2/1 -> Calculation  F/3(x2)
  a14/1 -> Calculation  F/7(c3)
  a15/1 -> Calculation  F/8(a1)
  a16/1 -> Calculation  F/9(a2)
  a17/1 -> Calculation  F/10(a3)
  a19/1 -> Calculation  F/12(f0)
  a18/1 -> Calculation  F/11(k)
  a13/1 -> Calculation  F/6(c2)
  a11/1 -> Calculation  F/5(c1)
  Calculation  F/1(F) -> Ftra/1
  z/1 -> Calculation  F/4(z)
  x1/1 -> Calculation  F/2(x1)
  I/1 -> Calculation  F/1(I)

== system RC_model_iden/Subsystem8/Subsystem ==
  x1 : Inport
  Constant : Constant  Value=a
  Constant1 : Constant  Value=b
  Delay : Delay  DelayLength=1  InitialCondition=0
  Delay1 : Delay  DelayLength=1  InitialCondition=0
  Delay2 : Delay  DelayLength=1  InitialCondition=0.17
  Delay3 : Delay  DelayLength=1  InitialCondition=0
  MATLAB Function : MATLAB Function  TreatAsAtomicUnit=on
  z : Outport  VectorParamsAs1DForOutWhenUnconnected=off
  wires:
  Delay3/1 -> MATLAB Function/6(x0)
  MATLAB Function/3(x01) -> Delay3/1
  Delay2/1 -> MATLAB Function/7(S0)
  MATLAB Function/4(S01) -> Delay2/1
  Delay1/1 -> MATLAB Function/5(x1k1)
  MATLAB Function/2(x1k2) -> Delay1/1
  Delay/1 -> MATLAB Function/4(zk1)
  MATLAB Function/1(zk) -> z/1, Delay/1
  Constant1/1 -> MATLAB Function/2(b)
  Constant/1 -> MATLAB Function/1(a)
  x1/1 -> MATLAB Function/3(x1k)

== system RC_model_iden/Subsystem9/Ftra ==
  I : Inport
  x1 : Inport  Port=2
  x2 : Inport  Port=3
  z : Inport  Port=4
  Calculation  F : MATLAB Function  TreatAsAtomicUnit=on
  a11 : Constant  Value=c1  SampleTime=-1
  a13 : Constant  Value=c2  SampleTime=-1
  a14 : Constant  Value=c3  SampleTime=-1
  a15 : Constant  Value=a1  SampleTime=-1
  a16 : Constant  Value=a2  SampleTime=-1
  a17 : Constant  Value=a3  SampleTime=-1
  a18 : Constant  Value=k  SampleTime=-1
  a19 : Constant  Value=f0  SampleTime=-1
  Ftra : Outport  VectorParamsAs1DForOutWhenUnconnected=off
  wires:
  x2/1 -> Calculation  F/3(x2)
  a14/1 -> Calculation  F/7(c3)
  a15/1 -> Calculation  F/8(a1)
  a16/1 -> Calculation  F/9(a2)
  a17/1 -> Calculation  F/10(a3)
  a19/1 -> Calculation  F/12(f0)
  a18/1 -> Calculation  F/11(k)
  a13/1 -> Calculation  F/6(c2)
  a11/1 -> Calculation  F/5(c1)
  Calculation  F/1(F) -> Ftra/1
  z/1 -> Calculation  F/4(z)
  x1/1 -> Calculation  F/2(x1)
  I/1 -> Calculation  F/1(I)

== system RC_model_iden/Subsystem9/Subsystem ==
  x1 : Inport
  Constant : Constant  Value=a
  Constant1 : Constant  Value=b
  Delay : Delay  DelayLength=1  InitialCondition=0
  Delay1 : Delay  DelayLength=1  InitialCondition=0
  Delay2 : Delay  DelayLength=1  InitialCondition=0.17
  Delay3 : Delay  DelayLength=1  InitialCondition=0
  MATLAB Function : MATLAB Function  TreatAsAtomicUnit=on
  z : Outport  VectorParamsAs1DForOutWhenUnconnected=off
  wires:
  Delay3/1 -> MATLAB Function/6(x0)
  MATLAB Function/3(x01) -> Delay3/1
  Delay2/1 -> MATLAB Function/7(S0)
  MATLAB Function/4(S01) -> Delay2/1
  Delay1/1 -> MATLAB Function/5(x1k1)
  MATLAB Function/2(x1k2) -> Delay1/1
  Delay/1 -> MATLAB Function/4(zk1)
  MATLAB Function/1(zk) -> z/1, Delay/1
  Constant1/1 -> MATLAB Function/2(b)
  Constant/1 -> MATLAB Function/1(a)
  x1/1 -> MATLAB Function/3(x1k)

== matlab function RC_model_iden/Subsystem2/Subsystem/MATLAB Function ==
  data: a input; zk output; b input; x1k input; zk1 input; x1k1 input; x0 input; S0 input; x1k2 output; x01 output; S01 output
function [zk,x1k2,x01,S01]= fcn(a,b,x1k,zk1,x1k1,x0,S0)


aal=S0*(x1k-x1k1);
    if x1k>x1k1;
        if aal<0;
            S0=(-log((1-zk1)/2)*a)^(1/b);
            x0=x1k1;
            S1=S0+x1k-x0;
        else
            S1=S0+x1k-x0;
        end
        
    elseif x1k<x1k1;
        if aal<0;
            S0=-(abs(log((1+zk1)/2)*a))^(1/b);
            x0=x1k1;
            S1=S0+x1k1-x0;
        else
            S1=S0+x1k1-x0;
        end
    else
        S1=S0+x1k-x0;
    end
       
    if S1>0
        zk=1-2*exp(-S1^b/a);
    else
        zk=-1+2*exp(-(abs(S1))^b/a);
    end
    x1k2=x1k;
    x01=x0;S01=S0;
end

== matlab function RC_model_iden/Subsystem3/Ftra/Calculation  F ==
  data: I input; x1 input; x2 input; z input; c1 input; c2 input; c3 input; F output; a1 input; a2 input; a3 input; k input; f0 input
function F = fcn(I,x1,x2,z,c1,c2,c3,a1,a2,a3,k,f0)
%#codegen



F=(c1*I^2+c2*I+c3)*x2+k*x1+(a1*I^2+a2*I+a3)*z+f0;
end

== matlab function RC_model_iden/Subsystem3/Subsystem/MATLAB Function ==
  data: a input; zk output; b input; x1k input; zk1 input; x1k1 input; x0 input; S0 input; x1k2 output; x01 output; S01 output
function [zk,x1k2,x01,S01]= fcn(a,b,x1k,zk1,x1k1,x0,S0)


aal=S0*(x1k-x1k1);
    if x1k>x1k1;
        if aal<0;
            S0=(-log((1-zk1)/2)*a)^(1/b);
            x0=x1k1;
            S1=S0+x1k-x0;
        else
            S1=S0+x1k-x0;
        end
        
    elseif x1k<x1k1;
        if aal<0;
            S0=-(abs(log((1+zk1)/2)*a))^(1/b);
            x0=x1k1;
            S1=S0+x1k1-x0;
        else
            S1=S0+x1k1-x0;
        end
    else
        S1=S0+x1k-x0;
    end
       
    if S1>0
        zk=1-2*exp(-S1^b/a);
    else
        zk=-1+2*exp(-(abs(S1))^b/a);
    end
    x1k2=x1k;
    x01=x0;S01=S0;
end

== matlab function RC_model_iden/Subsystem4/Ftra/Calculation  F ==
  data: I input; x1 input; x2 input; z input; c1 input; c2 input; c3 input; F output; a1 input; a2 input; a3 input; k input; f0 input
function F = fcn(I,x1,x2,z,c1,c2,c3,a1,a2,a3,k,f0)
%#codegen



F=(c1*I^2+c2*I+c3)*x2+k*x1+(a1*I^2+a2*I+a3)*z+f0;
end

== matlab function RC_model_iden/Subsystem4/Subsystem/MATLAB Function ==
  data: a input; zk output; b input; x1k input; zk1 input; x1k1 input; x0 input; S0 input; x1k2 output; x01 output; S01 output
function [zk,x1k2,x01,S01]= fcn(a,b,x1k,zk1,x1k1,x0,S0)


aal=S0*(x1k-x1k1);
    if x1k>x1k1;
        if aal<0;
            S0=(-log((1-zk1)/2)*a)^(1/b);
            x0=x1k1;
            S1=S0+x1k-x0;
        else
            S1=S0+x1k-x0;
        end
        
    elseif x1k<x1k1;
        if aal<0;
            S0=-(abs(log((1+zk1)/2)*a))^(1/b);
            x0=x1k1;
            S1=S0+x1k1-x0;
        else
            S1=S0+x1k1-x0;
        end
    else
        S1=S0+x1k-x0;
    end
       
    if S1>0
        zk=1-2*exp(-S1^b/a);
    else
        zk=-1+2*exp(-(abs(S1))^b/a);
    end
    x1k2=x1k;
    x01=x0;S01=S0;
end

== matlab function RC_model_iden/Subsystem7/Ftra/Calculation  F ==
  data: I input; x1 input; x2 input; z input; c1 input; c2 input; c3 input; F output; a1 input; a2 input; a3 input; k input; f0 input
function F = fcn(I,x1,x2,z,c1,c2,c3,a1,a2,a3,k,f0)
%#codegen


F=(c1*I^2+c2*I+c3)*x2+k*x1+(a1*I^2+a2*I+a3)*z+f0;
%F=c3*x2+k*x1+a3*z+f0;
end

== matlab function RC_model_iden/Subsystem5/Ftra/Calculation  F ==
  data: I input; x1 input; x2 input; z input; c1 input; c2 input; c3 input; F output; a1 input; a2 input; a3 input; k input; f0 input
function F = fcn(I,x1,x2,z,c1,c2,c3,a1,a2,a3,k,f0)
%#codegen



F=(c1*I^2+c2*I+c3)*x2+k*x1+(a1*I^2+a2*I+a3)*z+f0;
end

== matlab function RC_model_iden/Subsystem5/Subsystem/MATLAB Function ==
  data: a input; zk output; b input; x1k input; zk1 input; x1k1 input; x0 input; S0 input; x1k2 output; x01 output; S01 output
function [zk,x1k2,x01,S01]= fcn(a,b,x1k,zk1,x1k1,x0,S0)


aal=S0*(x1k-x1k1);
    if x1k>x1k1;
        if aal<0;
            S0=(-log((1-zk1)/2)*a)^(1/b);
            x0=x1k1;
            S1=S0+x1k-x0;
        else
            S1=S0+x1k-x0;
        end
        
    elseif x1k<x1k1;
        if aal<0;
            S0=-(abs(log((1+zk1)/2)*a))^(1/b);
            x0=x1k1;
            S1=S0+x1k1-x0;
        else
            S1=S0+x1k1-x0;
        end
    else
        S1=S0+x1k-x0;
    end
       
    if S1>0
        zk=1-2*exp(-S1^b/a);
    else
        zk=-1+2*exp(-(abs(S1))^b/a);
    end
    x1k2=x1k;
    x01=x0;S01=S0;
end

== matlab function RC_model_iden/Subsystem6/Ftra/Calculation  F ==
  data: I input; x1 input; x2 input; z input; c1 input; c2 input; c3 input; F output; a1 input; a2 input; a3 input; k input; f0 input
function F = fcn(I,x1,x2,z,c1,c2,c3,a1,a2,a3,k,f0)
%#codegen



F=(c1*I^2+c2*I+c3)*x2+k*x1+(a1*I^2+a2*I+a3)*z+f0;
end

== matlab function RC_model_iden/Subsystem6/Subsystem/MATLAB Function ==
  data: a input; zk output; b input; x1k input; zk1 input; x1k1 input; x0 input; S0 input; x1k2 output; x01 output; S01 output
function [zk,x1k2,x01,S01]= fcn(a,b,x1k,zk1,x1k1,x0,S0)


aal=S0*(x1k-x1k1);
    if x1k>x1k1;
        if aal<0;
            S0=(-log((1-zk1)/2)*a)^(1/b);
            x0=x1k1;
            S1=S0+x1k-x0;
        else
            S1=S0+x1k-x0;
        end
        
    elseif x1k<x1k1;
        if aal<0;
            S0=-(abs(log((1+zk1)/2)*a))^(1/b);
            x0=x1k1;
            S1=S0+x1k1-x0;
        else
            S1=S0+x1k1-x0;
        end
    else
        S1=S0+x1k-x0;
    end
       
    if S1>0
        zk=1-2*exp(-S1^b/a);
    else
        zk=-1+2*exp(-(abs(S1))^b/a);
    end
    x1k2=x1k;
    x01=x0;S01=S0;
end

== matlab function RC_model_iden/Subsystem8/Ftra/Calculation  F ==
  data: I input; x1 input; x2 input; z input; c1 input; c2 input; c3 input; F output; a1 input; a2 input; a3 input; k input; f0 input
function F = fcn(I,x1,x2,z,c1,c2,c3,a1,a2,a3,k,f0)
%#codegen



F=(c1*I^2+c2*I+c3)*x2+k*x1+(a1*I^2+a2*I+a3)*z+f0;
end

== matlab function RC_model_iden/Subsystem8/Subsystem/MATLAB Function ==
  data: a input; zk output; b input; x1k input; zk1 input; x1k1 input; x0 input; S0 input; x1k2 output; x01 output; S01 output
function [zk,x1k2,x01,S01]= fcn(a,b,x1k,zk1,x1k1,x0,S0)


aal=S0*(x1k-x1k1);
    if x1k>x1k1;
        if aal<0;
            S0=(-log((1-zk1)/2)*a)^(1/b);
            x0=x1k1;
            S1=S0+x1k-x0;
        else
            S1=S0+x1k-x0;
        end
        
    elseif x1k<x1k1;
        if aal<0;
            S0=-(abs(log((1+zk1)/2)*a))^(1/b);
            x0=x1k1;
            S1=S0+x1k1-x0;
        else
            S1=S0+x1k1-x0;
        end
    else
        S1=S0+x1k-x0;
    end
       
    if S1>0
        zk=1-2*exp(-S1^b/a);
    else
        zk=-1+2*exp(-(abs(S1))^b/a);
    end
    x1k2=x1k;
    x01=x0;S01=S0;
end

== matlab function RC_model_iden/Subsystem9/Ftra/Calculation  F ==
  data: I input; x1 input; x2 input; z input; c1 input; c2 input; c3 input; F output; a1 input; a2 input; a3 input; k input; f0 input
function F = fcn(I,x1,x2,z,c1,c2,c3,a1,a2,a3,k,f0)
%#codegen



F=(c1*I^2+c2*I+c3)*x2+k*x1+(a1*I^2+a2*I+a3)*z+f0;
end

== matlab function RC_model_iden/Subsystem9/Subsystem/MATLAB Function ==
  data: a input; zk output; b input; x1k input; zk1 input; x1k1 input; x0 input; S0 input; x1k2 output; x01 output; S01 output
function [zk,x1k2,x01,S01]= fcn(a,b,x1k,zk1,x1k1,x0,S0)


aal=S0*(x1k-x1k1);
    if x1k>x1k1;
        if aal<0;
            S0=(-log((1-zk1)/2)*a)^(1/b);
            x0=x1k1;
            S1=S0+x1k-x0;
        else
            S1=S0+x1k-x0;
        end
        
    elseif x1k<x1k1;
        if aal<0;
            S0=-(abs(log((1+zk1)/2)*a))^(1/b);
            x0=x1k1;
            S1=S0+x1k1-x0;
        else
            S1=S0+x1k1-x0;
        end
    else
        S1=S0+x1k-x0;
    end
       
    if S1>0
        zk=1-2*exp(-S1^b/a);
    else
        zk=-1+2*exp(-(abs(S1))^b/a);
    end
    x1k2=x1k;
    x01=x0;S01=S0;
end

== matlab function RC_model_iden/Subsystem10/Ftra/Calculation  F ==
  data: I input; x1 input; x2 input; z input; c1 input; c2 input; c3 input; F output; a1 input; a2 input; a3 input; k input; f0 input
function F = fcn(I,x1,x2,z,c1,c2,c3,a1,a2,a3,k,f0)
%#codegen



F=(c1*I^2+c2*I+c3)*x2+k*x1+(a1*I^2+a2*I+a3)*z+f0;
end

== matlab function RC_model_iden/Subsystem10/Subsystem/MATLAB Function ==
  data: a input; zk output; b input; x1k input; zk1 input; x1k1 input; x0 input; S0 input; x1k2 output; x01 output; S01 output
function [zk,x1k2,x01,S01]= fcn(a,b,x1k,zk1,x1k1,x0,S0)


aal=S0*(x1k-x1k1);
    if x1k>x1k1;
        if aal<0;
            S0=(-log((1-zk1)/2)*a)^(1/b);
            x0=x1k1;
            S1=S0+x1k-x0;
        else
            S1=S0+x1k-x0;
        end
        
    elseif x1k<x1k1;
        if aal<0;
            S0=-(abs(log((1+zk1)/2)*a))^(1/b);
            x0=x1k1;
            S1=S0+x1k1-x0;
        else
            S1=S0+x1k1-x0;
        end
    else
        S1=S0+x1k-x0;
    end
       
    if S1>0
        zk=1-2*exp(-S1^b/a);
    else
        zk=-1+2*exp(-(abs(S1))^b/a);
    end
    x1k2=x1k;
    x01=x0;S01=S0;
end

== matlab function RC_model_iden/Subsystem11/Ftra/Calculation  F ==
  data: I input; x1 input; x2 input; z input; c1 input; c2 input; c3 input; F output; a1 input; a2 input; a3 input; k input; f0 input
function F = fcn(I,x1,x2,z,c1,c2,c3,a1,a2,a3,k,f0)
%#codegen



F=(c1*I^2+c2*I+c3)*x2+k*x1+(a1*I^2+a2*I+a3)*z+f0;
end

== matlab function RC_model_iden/Subsystem7/Subsystem/MATLAB Function ==
  data: a input; zk output; b input; x1k input; zk1 input; x1k1 input; x0 input; S0 input; x1k2 output; x01 output; S01 output
function [zk,x1k2,x01,S01]= fcn(a,b,x1k,zk1,x1k1,x0,S0)


aal=S0*(x1k-x1k1);
    if x1k>x1k1;
        if aal<0;
            S0=(-log((1-zk1)/2)*a)^(1/b);
            x0=x1k1;
            S1=S0+x1k-x0;
        else
            S1=S0+x1k-x0;
        end
        
    elseif x1k<x1k1;
        if aal<0;
            S0=-(abs(log((1+zk1)/2 )*a))^(1/b);
            x0=x1k1;
            S1=S0+x1k1-x0;
        else
            S1=S0+x1k1-x0;
        end
    else
        S1=S0+x1k-x0;
    end
       
    if S1>0
        zk=1-2*exp(-S1^b/a);
    else
        zk=-1+2*exp(-(abs(S1))^b/a);
    end
    x1k2=x1k;
    x01=x0;S01=S0;
end

== matlab function RC_model_iden/Subsystem11/Subsystem/MATLAB Function ==
  data: a input; zk output; b input; x1k input; zk1 input; x1k1 input; x0 input; S0 input; x1k2 output; x01 output; S01 output
function [zk,x1k2,x01,S01]= fcn(a,b,x1k,zk1,x1k1,x0,S0)


aal=S0*(x1k-x1k1);
    if x1k>x1k1;
        if aal<0;
            S0=(-log((1-zk1)/2)*a)^(1/b);
            x0=x1k1;
            S1=S0+x1k-x0;
        else
            S1=S0+x1k-x0;
        end
        
    elseif x1k<x1k1;
        if aal<0;
            S0=-(abs(log((1+zk1)/2)*a))^(1/b);
            x0=x1k1;
            S1=S0+x1k1-x0;
        else
            S1=S0+x1k1-x0;
        end
    else
        S1=S0+x1k-x0;
    end
       
    if S1>0
        zk=1-2*exp(-S1^b/a);
    else
        zk=-1+2*exp(-(abs(S1))^b/a);
    end
    x1k2=x1k;
    x01=x0;S01=S0;
end

== matlab function RC_model_iden/Subsystem1/Ftra/Calculation  F ==
  data: I input; x1 input; x2 input; z input; c1 input; c2 input; c3 input; F output; a1 input; a2 input; a3 input; k input; f0 input
function F = fcn(I,x1,x2,z,c1,c2,c3,a1,a2,a3,k,f0)
%#codegen



F=(c1*I^2+c2*I+c3)*x2+k*x1+(a1*I^2+a2*I+a3)*z+f0;
end

== matlab function RC_model_iden/Subsystem1/Subsystem/MATLAB Function ==
  data: a input; zk output; b input; x1k input; zk1 input; x1k1 input; x0 input; S0 input; x1k2 output; x01 output; S01 output
function [zk,x1k2,x01,S01]= fcn(a,b,x1k,zk1,x1k1,x0,S0)


aal=S0*(x1k-x1k1);
    if x1k>x1k1;
        if aal<0;
            S0=(-log((1-zk1)/2)*a)^(1/b);
            x0=x1k1;
            S1=S0+x1k-x0;
        else
            S1=S0+x1k-x0;
        end
        
    elseif x1k<x1k1;
        if aal<0;
            S0=-(abs(log((1+zk1)/2)*a))^(1/b);
            x0=x1k1;
            S1=S0+x1k1-x0;
        else
            S1=S0+x1k1-x0;
        end
    else
        S1=S0+x1k-x0;
    end
       
    if S1>0
        zk=1-2*exp(-S1^b/a);
    else
        zk=-1+2*exp(-(abs(S1))^b/a);
    end
    x1k2=x1k;
    x01=x0;S01=S0;
end

== matlab function RC_model_iden/Subsystem2/Ftra/Calculation  F ==
  data: I input; x1 input; x2 input; z input; c1 input; c2 input; c3 input; F output; a1 input; a2 input; a3 input; k0 input; f0 input
function F = fcn(I,x1,x2,z,c1,c2,c3,a1,a2,a3,k0,f0)
%#codegen



F=(c1*I^2+c2*I+c3)*x2+k0*x1+(a1*I^2+a2*I+a3)*z+f0;
end
